simulink model "mech_motorcycle_stability"  (Simulink 7.1)
settings: Solver=ode45  StartTime=0.0  StopTime=3  RelTol=1e-3  AbsTol=1e-6
PreLoadFcn:
  | vu=53;mech_motorcycle_data
values from neighbouring files (symbols this model uses):
  Cf1 = -13.25+1.302*Zf-(1.39e-4)*Zf^2    [mech_motorcycle_data.m]
  Cf2 = 2.788+0.0165*Zf+(3.9e-6)*Zf^2    [mech_motorcycle_data.m]
  Cf3 = -0.06*Zf    [mech_motorcycle_data.m]
  Cfvf = -300+28.577*Zf-0.0143*Zf^2+(1.431e-6)*Zf^3+(3.347e-10)*Zf^4    [mech_motorcycle_data.m]
  Cfvr = -92.9+23.129*Zr-(4.663/1000)*Zr^2-(6.457e-7)*Zr^3+(1.887e-10)*Zr^4    [mech_motorcycle_data.m]
  Cmvf = -0.281+0.2442*Zf+(8.575e-5)*Zf^2    [mech_motorcycle_data.m]
  Cmvr = 9+0.3573*Zr + (3.378e-5)*Zr^2    [mech_motorcycle_data.m]
  Cr1 = 27.38+0.9727*Zr-(4e-6)*Zr^2    [mech_motorcycle_data.m]
  Cr2 = 2.056+0.01282*Zr+(4.928e-6)*Zr^2    [mech_motorcycle_data.m]
  Cr3 = -0.07*Zr    [mech_motorcycle_data.m]
  D = inv(D)    [mech_stewart_MV_controller.m]    (also in mech_stewart_control_Hinf.mat = [-0.999999999853 7.5115525316e-12 1.21216792902e-05 1.919374)
  epsilon = 0.47    [mech_motorcycle_data.m]    (also in mech_motorcycle_data_nonlinear.m = 0.52)
  epsilon1 = 1.435    [mech_motorcycle_data.m]
  G = 9.81    [mech_motorcycle_data.m]    (also in mech_sceng_init.m = 1.4)
  Mfw = 0    [mech_motorcycle_data.m]    (also in mech_motorcycle_data_nonlinear.m = 25.6)
  Mrw = 0    [mech_motorcycle_data.m]    (also in mech_motorcycle_data_nonlinear.m = 25.6)
  Rf = 0.336    [mech_motorcycle_data.m]
  Rr = 0.321    [mech_motorcycle_data.m]
  sigmaf = 0.1012+(1.297e-4)*Zf-(3.267e-8)*Zf^2    [mech_motorcycle_data.m]
  sigmar = 0.03594+(1.941e-4)*Zr-(5.667e-8)*Zr^2+(5.728e-12)*Zr^3    [mech_motorcycle_data.m]
  Zf = ((Mf.value*(bb+kk)+Mr.value*bb+Mb.value*(bb-bb_b)+Mp.value*(bb-bb_p))*G-(vu^2)*(Dc.value*hh_cp+Lc.value*whl_bs/2))/whl_bs    [mech_motorcycle_data.m]
  Zr = (Mf.value+Mr.value+Mp.value+Mb.value)*G-Lc.value*vu^2-Zf    [mech_motorcycle_data.m]
undefined symbols (not defined in the file or in its folder): Crr1, Crr2, D_gamma, D_lamda, D_steer, D_v, D_zita, Dc, ifwy, Ifx, Ifxz, Ifz, Ipx, Ipxz, Ipz, irwx, irwy, Irx, Irxz, iry, Irz, k_gamma, k_lamda, k_steer, k_v, k_zita, Lc, m, Mb, Mf, Mp, Mr, rad, s
libraries: mblibv1 x43
(part 2 of 2)

== system mech_motorcycle_stability/Twist spring-damper ==
  note: Twist spring damper model
  note: Press any key to continue
  Damping : Gain  Gain=-D_lamda.value  ParameterDataType=sfix(16)  ParameterScaling=2^0  OutDataType=sfix(16)  OutScaling=2^0  SaturateOnIntegerOverflow=on  OutDataTypeStr=Inherit: Same as input  ParamDataTypeStr=Inherit: Same as input
  Demux : Demux  Outputs=2
  Initial Force : Constant  Value=0  OutDataType=sfix(16)  OutScaling=2^0
  Joint Actuator : mblibv1/Sensors &  Actuators/Joint Actuator  DialogController=MECH.DynMechDlgSource  SystemSampleTime=-1  PhysicalDomain=Mechanical  PortType=blob  ActuationStyle=Force  AngleUnits=rad  ArcVelocityUnits=rad/s  ArcAccelerationUnits=rad/s^2  CoordPositionUnits=m  VelocityUnits=m/s  AccelerationUnits=m/s^2  ForceUnits=N  TorqueUnits=N-m  ActiveIO=on  Width=1  DialogClass=MechanicalActuatorBlock  Primitive=R1  ReferenceFrame=Absolute (INERTIAL)
  Joint Sensor : mblibv1/Sensors &  Actuators/Joint Sensor  DialogController=MECH.DynMechDlgSource  SystemSampleTime=-1  PhysicalDomain=Mechanical  PortType=blob  Muxed=on  Pose=off  Angle=on  AngleUnits=rad  ArcVelocity=on  ArcVelocityUnits=rad/s  ArcAcceleration=off  ArcAccelerationUnits=deg/s^2  CoordPosition=on  CoordPositionUnits=m  Velocity=on  VelocityUnits=m/s  Acceleration=off  AccelerationUnits=m/s^2  Quaternion=on  QuaternionDT=off  QuaternionDDT=off  QuaternionUnits=off  OutputVector=[ 1 1 ]  ActiveIO=on  Width=2  DialogClass=MechanicalSensorBlock  Primitive=R1  Force=off  ForceUnits=N  Torque=off  TorqueUnits=N-m  ReferenceFrame=Absolute (INERTIAL)  ReactionSensedSide=Base  ReactionReferenceFrame=Absolute (World)  ReactionForce=off  ReactionForceUnits=N  ReactionMoment=off  ReactionMomentUnits=N-m
  Stiffness : Gain  Gain=-k_lamda.value  ParameterDataType=sfix(16)  ParameterScaling=2^0  OutDataType=sfix(16)  OutScaling=2^0  SaturateOnIntegerOverflow=on  OutDataTypeStr=Inherit: Same as input  ParamDataTypeStr=Inherit: Same as input
  Sum : Sum  Inputs=+++  OutDataType=sfix(16)  OutScaling=2^0  SaturateOnIntegerOverflow=on  InputSameDT=on  OutDataTypeStr=Inherit: Same as first input
  S : PMIOPort  Port=1  Side=Left
  A : PMIOPort  Orientation=left  Port=2  Side=Right
  wires:
  Sum/1 -> Joint Actuator/1  "Torque (Nm)"
  Joint Sensor/1 -> Demux/1
  Demux/1 -> Stiffness/1  "Angle (rad)"
  Demux/2 -> Damping/1  "Angular velocity (rad/s)"
  Damping/1 -> Sum/2
  Stiffness/1 -> Sum/1
  Initial Force/1 -> Sum/3
  connections:
  S/RConn1 -- Joint Sensor/LConn1
  Joint Actuator/RConn1 -- A/RConn1

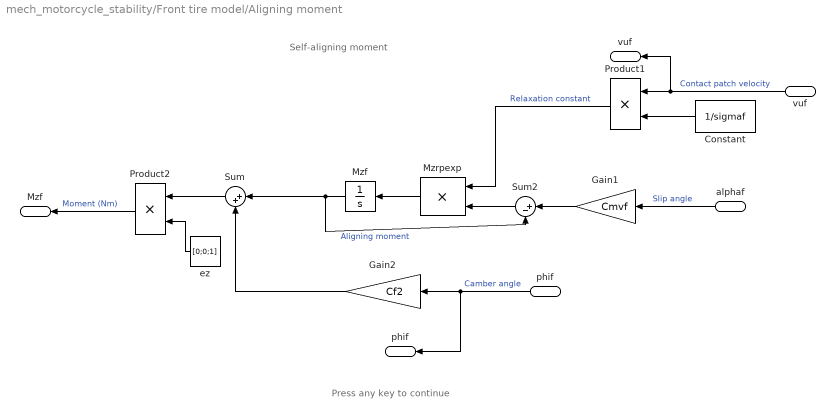
== system mech_motorcycle_stability/Front tire model/Aligning moment ==
  note: Self-aligning moment
  note: Press any key to continue
  vuf : Inport  Orientation=left  OutDataType=sfix(16)  OutScaling=2^0
  phif : Inport  Orientation=left  Port=2  OutDataType=sfix(16)  OutScaling=2^0
  alphaf : Inport  Orientation=left  Port=3  OutDataType=sfix(16)  OutScaling=2^0
  Constant : Constant  Orientation=left  Value=1/sigmaf  OutDataType=sfix(16)  OutScaling=2^0
  Gain1 : Gain  Orientation=left  Gain=Cmvf  ParameterDataType=sfix(16)  ParameterScaling=2^0  OutDataType=sfix(16)  OutScaling=2^0  SaturateOnIntegerOverflow=on  OutDataTypeStr=Inherit: Same as input  ParamDataTypeStr=Inherit: Same as input
  Gain2 : Gain  Orientation=left  Gain=Cf2  ParameterDataType=sfix(16)  ParameterScaling=2^0  OutDataType=sfix(16)  OutScaling=2^0  SaturateOnIntegerOverflow=on  OutDataTypeStr=Inherit: Same as input  ParamDataTypeStr=Inherit: Same as input
  "Mzf  " : Integrator  Orientation=left  ZeroCross=off
  Mzrpexp : Product  Orientation=left  OutDataType=sfix(16)  OutScaling=2^0  SaturateOnIntegerOverflow=on  InputSameDT=on  OutDataTypeStr=Inherit: Same as first input
  Product1 : Product  Orientation=left  OutDataType=sfix(16)  OutScaling=2^0  SaturateOnIntegerOverflow=on  InputSameDT=on  OutDataTypeStr=Inherit: Same as first input
  Product2 : Product  Orientation=left  OutDataType=sfix(16)  OutScaling=2^0  SaturateOnIntegerOverflow=on  InputSameDT=on  OutDataTypeStr=Inherit: Same as first input
  Sum : Sum  Orientation=left  Inputs=|++  OutDataType=sfix(16)  OutScaling=2^0  SaturateOnIntegerOverflow=on  InputSameDT=on  OutDataTypeStr=Inherit: Same as first input
  Sum2 : Sum  Orientation=left  Inputs=|+-  OutDataType=sfix(16)  OutScaling=2^0  SaturateOnIntegerOverflow=on  InputSameDT=on  OutDataTypeStr=Inherit: Same as first input
  ez : Constant  Orientation=left  Value=[0;0;1]  OutDataType=sfix(16)  OutScaling=2^0
  Mzf : Outport  Orientation=left  OutDataType=sfix(16)  OutScaling=2^0
  "phif " : Outport  Orientation=left  Port=2  OutDataType=sfix(16)  OutScaling=2^0
  "vuf " : Outport  Orientation=left  Port=3  OutDataType=sfix(16)  OutScaling=2^0
  wires:
  Product2/1 -> Mzf/1  "Moment (Nm)"
  ez/1 -> Product2/2
  Sum/1 -> Product2/1
  Gain2/1 -> Sum/2
  phif/1 -> "phif "/1, Gain2/1  "Camber angle"
  alphaf/1 -> Gain1/1  "Slip angle"
  "Mzf  "/1 -> Sum2/2, Sum/1  "Aligning moment"
  Gain1/1 -> Sum2/1
  Sum2/1 -> Mzrpexp/2
  Product1/1 -> Mzrpexp/1  "Relaxation constant"
  Mzrpexp/1 -> "Mzf  "/1
  Constant/1 -> Product1/2
  vuf/1 -> Product1/1, "vuf "/1  "Contact patch velocity"

== system mech_motorcycle_stability/Front tire model/Contact ==
  note: Contact
  note: Press any key to continue
  Body Sensor : mblibv1/Sensors &  Actuators/Body Sensor  Orientation=left  DialogController=MECH.DynMechDlgSource  SystemSampleTime=-1  PhysicalDomain=Mechanical  PortType=blob  Muxed=off  Pose=on  Angle=on  AngleUnits=deg  ArcVelocity=off  ArcVelocityUnits=rad/s  ArcAcceleration=off  ArcAccelerationUnits=rad/s^2  CoordPosition=off  CoordPositionUnits=m  Velocity=on  VelocityUnits=m/s  Acceleration=off  AccelerationUnits=m/s^2  Quaternion=on  QuaternionDT=off  QuaternionDDT=off  QuaternionUnits=off  OutputVector=[ 3 9 ]  ActiveIO=on  Width=12  DialogClass=MechanicalSensorBlock  ReferenceFrame=Absolute (World)
  Contact geometry : Subsystem  Orientation=left
  Product1 : Product  Orientation=left  Multiplication=Matrix(*)  OutDataType=sfix(16)  OutScaling=2^0  SaturateOnIntegerOverflow=on  InputSameDT=on  OutDataTypeStr=Inherit: Same as first input
  Reshape : Reshape  Orientation=left  OutputDimensionality=Row vector (2-D)
  Reshape1 : Reshape  Orientation=left  OutputDimensionality=Column vector (2-D)
  Rear Wheel : PMIOPort  Orientation=left  Port=1  Side=Left
  fw_long : Outport  Orientation=left  OutDataType=sfix(16)  OutScaling=2^0
  vuf : Outport  Orientation=left  Port=2  OutDataType=sfix(16)  OutScaling=2^0
  phif : Outport  Orientation=left  Port=3  OutDataType=sfix(16)  OutScaling=2^0
  dfwcp_dt : Outport  Orientation=left  Port=4  OutDataType=sfix(16)  OutScaling=2^0
  fw_lat : Outport  Orientation=left  Port=5  OutDataType=sfix(16)  OutScaling=2^0
  wires:
  Contact geometry/3(phif) -> phif/1  "Camber angle (rad)"
  Contact geometry/1(fw_lat) -> fw_lat/1  "Lateral direction"
  Body Sensor/2 -> Contact geometry/1(T)  "Body orientation"
  Reshape1/1 -> Product1/2
  Reshape/1 -> Product1/1
  Product1/1 -> vuf/1  "Longitudinal component (m/s)"
  Body Sensor/1 -> Reshape/1, dfwcp_dt/1  "Contact patch velocity (m/s)"
  Contact geometry/2(fw_long) -> fw_long/1, Reshape1/1  "Longitudinal direction"
  connections:
  Rear Wheel/RConn1 -- Body Sensor/LConn1

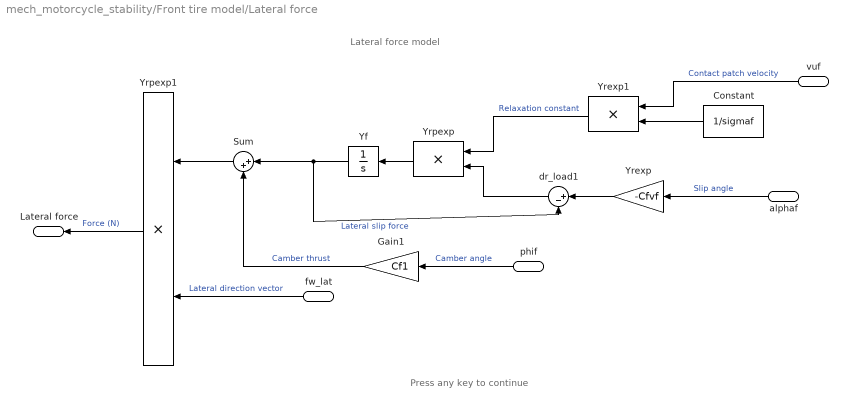
== system mech_motorcycle_stability/Front tire model/Lateral force ==
  note: Lateral force model
  note: Press any key to continue
  phif : Inport  Orientation=left  OutDataType=sfix(16)  OutScaling=2^0
  vuf : Inport  Orientation=left  Port=2  OutDataType=sfix(16)  OutScaling=2^0
  alphaf : Inport  Orientation=left  Port=3  OutDataType=sfix(16)  OutScaling=2^0
  fw_lat : Inport  Orientation=left  Port=4  OutDataType=sfix(16)  OutScaling=2^0
  Constant : Constant  Orientation=left  Value=1/sigmaf  OutDataType=sfix(16)  OutScaling=2^0
  Gain1 : Gain  Orientation=left  Gain=Cf1  ParameterDataType=sfix(16)  ParameterScaling=2^0  OutDataType=sfix(16)  OutScaling=2^0  SaturateOnIntegerOverflow=on  OutDataTypeStr=Inherit: Same as input  ParamDataTypeStr=Inherit: Same as input
  Sum : Sum  Orientation=left  Inputs=|++  OutDataType=sfix(16)  OutScaling=2^0  SaturateOnIntegerOverflow=on  InputSameDT=on  OutDataTypeStr=Inherit: Same as first input
  Yf : Integrator  Orientation=left  ZeroCross=off
  Yrexp : Gain  Orientation=left  Gain=-Cfvf  ParameterDataType=sfix(16)  ParameterScaling=2^0  OutDataType=sfix(16)  OutScaling=2^0  SaturateOnIntegerOverflow=on  OutDataTypeStr=Inherit: Same as input  ParamDataTypeStr=Inherit: Same as input
  Yrexp1 : Product  Orientation=left  OutDataType=sfix(16)  OutScaling=2^0  SaturateOnIntegerOverflow=on  InputSameDT=on  OutDataTypeStr=Inherit: Same as first input
  Yrpexp : Product  Orientation=left  OutDataType=sfix(16)  OutScaling=2^0  SaturateOnIntegerOverflow=on  InputSameDT=on  OutDataTypeStr=Inherit: Same as first input
  Yrpexp1 : Product  Orientation=left  OutDataType=sfix(16)  OutScaling=2^0  SaturateOnIntegerOverflow=on  InputSameDT=on  OutDataTypeStr=Inherit: Same as first input
  dr_load1 : Sum  Orientation=left  Inputs=|+-  OutDataType=sfix(16)  OutScaling=2^0  SaturateOnIntegerOverflow=on  InputSameDT=on  OutDataTypeStr=Inherit: Same as first input
  Lateral force : Outport  Orientation=left  OutDataType=sfix(16)  OutScaling=2^0
  wires:
  Yrpexp1/1 -> Lateral force/1  "Force (N)"
  fw_lat/1 -> Yrpexp1/2  "Lateral direction vector"
  Sum/1 -> Yrpexp1/1
  Gain1/1 -> Sum/2  "Camber thrust"
  phif/1 -> Gain1/1  "Camber angle"
  alphaf/1 -> Yrexp/1  "Slip angle"
  Yrexp/1 -> dr_load1/1
  Yf/1 -> Sum/1, dr_load1/2  "Lateral slip force"
  Yrpexp/1 -> Yf/1
  dr_load1/1 -> Yrpexp/2
  Yrexp1/1 -> Yrpexp/1  "Relaxation constant"
  Constant/1 -> Yrexp1/2
  vuf/1 -> Yrexp1/1  "Contact patch velocity"

== system mech_motorcycle_stability/Front tire model/Lateral slip computation ==
  note: Lateral slip computation
  note: Press any key to continue
  dfwcp_dt : Inport  Orientation=left  OutDataType=sfix(16)  OutScaling=2^0
  fw_lat : Inport  Orientation=left  Port=2  OutDataType=sfix(16)  OutScaling=2^0
  Fcn : Fcn  Orientation=left  Expr=1.0/sqrt(u[1]*u[1] + u[2]*u[2] + u[3]*u[3])
  Product : Product  Orientation=left  OutDataType=sfix(16)  OutScaling=2^0  SaturateOnIntegerOverflow=on  InputSameDT=on  OutDataTypeStr=Inherit: Same as first input
  Product1 : Product  Orientation=left  Multiplication=Matrix(*)  OutDataType=sfix(16)  OutScaling=2^0  SaturateOnIntegerOverflow=on  InputSameDT=on  OutDataTypeStr=Inherit: Same as first input
  Reshape : Reshape  Orientation=left  OutputDimensionality=Row vector (2-D)
  Reshape1 : Reshape  Orientation=left  OutputDimensionality=Column vector (2-D)
  Trigonometric Function : Trigonometry  Orientation=left  Operator=asin
  alphaf : Outport  Orientation=left  OutDataType=sfix(16)  OutScaling=2^0
  wires:
  Product/1 -> Reshape/1  "Unit vector"
  Fcn/1 -> Product/1
  dfwcp_dt/1 -> Fcn/1, Product/2  "Velocity (m/s)"
  fw_lat/1 -> Reshape1/1  "Lateral direction"
  Reshape1/1 -> Product1/2
  Trigonometric Function/1 -> alphaf/1  "Slip angle (rad)"
  Product1/1 -> Trigonometric Function/1
  Reshape/1 -> Product1/1

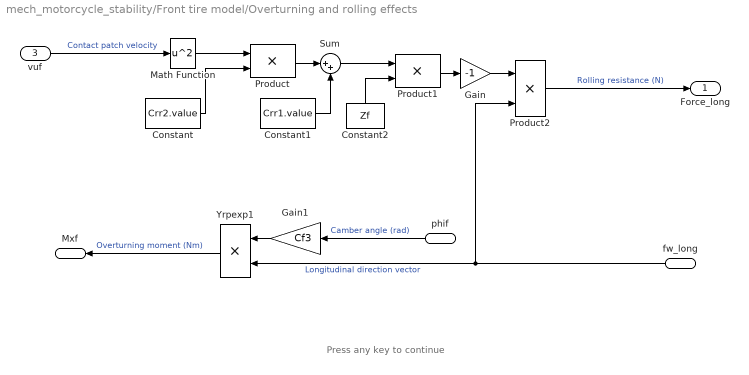
== system mech_motorcycle_stability/Front tire model/Overturning and rolling effects ==
  note: Press any key to continue
  fw_long : Inport  Orientation=left  OutDataType=sfix(16)  OutScaling=2^0
  phif : Inport  Orientation=left  Port=2  OutDataType=sfix(16)  OutScaling=2^0
  vuf : Inport  Port=3  OutDataType=sfix(16)  OutScaling=2^0
  Constant : Constant  Value=Crr2.value  OutDataType=sfix(16)  OutScaling=2^0
  Constant1 : Constant  Value=Crr1.value  OutDataType=sfix(16)  OutScaling=2^0
  Constant2 : Constant  Orientation=up  Value=Zf  OutDataType=sfix(16)  OutScaling=2^0
  Gain : Gain  Gain=-1  ParameterDataType=sfix(16)  ParameterScaling=2^0  OutDataType=sfix(16)  OutScaling=2^0  SaturateOnIntegerOverflow=on  OutDataTypeStr=Inherit: Same as input  ParamDataTypeStr=Inherit: Same as input
  Gain1 : Gain  Orientation=left  Gain=Cf3  ParameterDataType=sfix(16)  ParameterScaling=2^0  OutDataType=sfix(16)  OutScaling=2^0  SaturateOnIntegerOverflow=on  OutDataTypeStr=Inherit: Same as input  ParamDataTypeStr=Inherit: Same as input
  Math Function : Math  Operator=square  OutDataType=sfix(16)  OutScaling=2^0  SaturateOnIntegerOverflow=on
  Product : Product  OutDataType=sfix(16)  OutScaling=2^0  SaturateOnIntegerOverflow=on  InputSameDT=on  OutDataTypeStr=Inherit: Same as first input
  Product1 : Product  OutDataType=sfix(16)  OutScaling=2^0  SaturateOnIntegerOverflow=on  InputSameDT=on  OutDataTypeStr=Inherit: Same as first input
  Product2 : Product  OutDataType=sfix(16)  OutScaling=2^0  SaturateOnIntegerOverflow=on  InputSameDT=on  OutDataTypeStr=Inherit: Same as first input
  Sum : Sum  Inputs=|++  OutDataType=sfix(16)  OutScaling=2^0  SaturateOnIntegerOverflow=on  InputSameDT=on  OutDataTypeStr=Inherit: Same as first input
  Yrpexp1 : Product  Orientation=left  OutDataType=sfix(16)  OutScaling=2^0  SaturateOnIntegerOverflow=on  InputSameDT=on  OutDataTypeStr=Inherit: Same as first input
  Force_long : Outport  OutDataType=sfix(16)  OutScaling=2^0
  Mxf : Outport  Orientation=left  Port=2  OutDataType=sfix(16)  OutScaling=2^0
  wires:
  Yrpexp1/1 -> Mxf/1  "Overturning moment (Nm)"
  Gain1/1 -> Yrpexp1/1
  phif/1 -> Gain1/1  "Camber angle (rad)"
  Product2/1 -> Force_long/1  "Rolling resistance (N)"
  Gain/1 -> Product2/1
  Product1/1 -> Gain/1
  Constant2/1 -> Product1/2
  Sum/1 -> Product1/1
  Constant1/1 -> Sum/2
  Constant/1 -> Product/2
  Math Function/1 -> Product/1
  Product/1 -> Sum/1
  vuf/1 -> Math Function/1  "Contact patch velocity"
  fw_long/1 -> Yrpexp1/2, Product2/2  "Longitudinal direction vector"

== system mech_motorcycle_stability/Front tire model/Vertical force ==
  note: Press any key to continue
  Constant : Constant  Orientation=left  Value=-Zf  OutDataType=sfix(16)  OutScaling=2^0
  Product2 : Product  Orientation=left  OutDataType=sfix(16)  OutScaling=2^0  SaturateOnIntegerOverflow=on  InputSameDT=on  OutDataTypeStr=Inherit: Same as first input
  ez : Constant  Orientation=left  Value=[0;0;1]  OutDataType=sfix(16)  OutScaling=2^0
  Force_vert : Outport  Orientation=left  OutDataType=sfix(16)  OutScaling=2^0
  wires:
  ez/1 -> Product2/2
  Constant/1 -> Product2/1
  Product2/1 -> Force_vert/1  "Vertical force (N)"

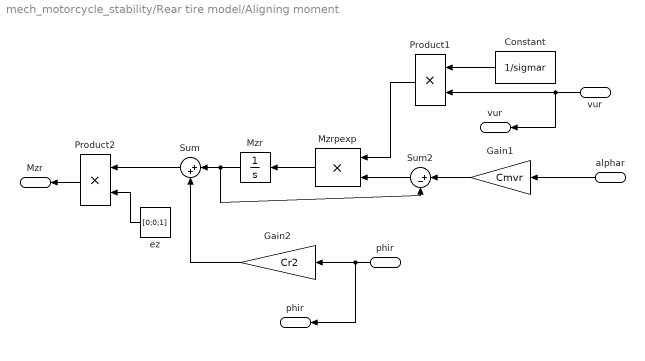
== system mech_motorcycle_stability/Rear tire model/Aligning moment ==
  vur : Inport  Orientation=left  OutDataType=sfix(16)  OutScaling=2^0
  phir : Inport  Orientation=left  Port=2  OutDataType=sfix(16)  OutScaling=2^0
  alphar : Inport  Orientation=left  Port=3  OutDataType=sfix(16)  OutScaling=2^0
  Constant : Constant  Orientation=left  Value=1/sigmar  OutDataType=sfix(16)  OutScaling=2^0
  Gain1 : Gain  Orientation=left  Gain=Cmvr  ParameterDataType=sfix(16)  ParameterScaling=2^0  OutDataType=sfix(16)  OutScaling=2^0  SaturateOnIntegerOverflow=on  OutDataTypeStr=Inherit: Same as input  ParamDataTypeStr=Inherit: Same as input
  Gain2 : Gain  Orientation=left  Gain=Cr2  ParameterDataType=sfix(16)  ParameterScaling=2^0  OutDataType=sfix(16)  OutScaling=2^0  SaturateOnIntegerOverflow=on  OutDataTypeStr=Inherit: Same as input  ParamDataTypeStr=Inherit: Same as input
  "Mzr  " : Integrator  Orientation=left  ZeroCross=off
  Mzrpexp : Product  Orientation=left  OutDataType=sfix(16)  OutScaling=2^0  SaturateOnIntegerOverflow=on  InputSameDT=on  OutDataTypeStr=Inherit: Same as first input
  Product1 : Product  Orientation=left  OutDataType=sfix(16)  OutScaling=2^0  SaturateOnIntegerOverflow=on  InputSameDT=on  OutDataTypeStr=Inherit: Same as first input
  Product2 : Product  Orientation=left  OutDataType=sfix(16)  OutScaling=2^0  SaturateOnIntegerOverflow=on  InputSameDT=on  OutDataTypeStr=Inherit: Same as first input
  Sum : Sum  Orientation=left  Inputs=|++  OutDataType=sfix(16)  OutScaling=2^0  SaturateOnIntegerOverflow=on  InputSameDT=on  OutDataTypeStr=Inherit: Same as first input
  Sum2 : Sum  Orientation=left  Inputs=|+-  OutDataType=sfix(16)  OutScaling=2^0  SaturateOnIntegerOverflow=on  InputSameDT=on  OutDataTypeStr=Inherit: Same as first input
  ez : Constant  Orientation=left  Value=[0;0;1]  OutDataType=sfix(16)  OutScaling=2^0
  Mzr : Outport  Orientation=left  OutDataType=sfix(16)  OutScaling=2^0
  "phir " : Outport  Orientation=left  Port=2  OutDataType=sfix(16)  OutScaling=2^0
  "vur " : Outport  Orientation=left  Port=3  OutDataType=sfix(16)  OutScaling=2^0
  wires:
  Mzrpexp/1 -> "Mzr  "/1
  Product1/1 -> Mzrpexp/1
  Sum2/1 -> Mzrpexp/2
  vur/1 -> Product1/2, "vur "/1
  Gain1/1 -> Sum2/1
  "Mzr  "/1 -> Sum2/2, Sum/1
  alphar/1 -> Gain1/1
  Constant/1 -> Product1/1
  phir/1 -> Gain2/1, "phir "/1
  Gain2/1 -> Sum/2
  Sum/1 -> Product2/1
  ez/1 -> Product2/2
  Product2/1 -> Mzr/1

== system mech_motorcycle_stability/Rear tire model/Contact ==
  Body Sensor : mblibv1/Sensors &  Actuators/Body Sensor  Orientation=left  DialogController=MECH.DynMechDlgSource  SystemSampleTime=-1  PhysicalDomain=Mechanical  PortType=blob  Muxed=off  Pose=on  Angle=on  AngleUnits=deg  ArcVelocity=off  ArcVelocityUnits=rad/s  ArcAcceleration=off  ArcAccelerationUnits=rad/s^2  CoordPosition=off  CoordPositionUnits=m  Velocity=on  VelocityUnits=m/s  Acceleration=off  AccelerationUnits=m/s^2  Quaternion=on  QuaternionDT=off  QuaternionDDT=off  QuaternionUnits=off  OutputVector=[ 3 9 ]  ActiveIO=on  Width=12  DialogClass=MechanicalSensorBlock  ReferenceFrame=Absolute (World)
  Contact geometry : Subsystem  Orientation=left
  Product1 : Product  Orientation=left  Multiplication=Matrix(*)  OutDataType=sfix(16)  OutScaling=2^0  SaturateOnIntegerOverflow=on  InputSameDT=on  OutDataTypeStr=Inherit: Same as first input
  Reshape : Reshape  Orientation=left  OutputDimensionality=Row vector (2-D)
  Reshape1 : Reshape  Orientation=left  OutputDimensionality=Column vector (2-D)
  Rear Wheel : PMIOPort  Orientation=left  Port=1  Side=Left
  rw_long : Outport  Orientation=left  OutDataType=sfix(16)  OutScaling=2^0
  vur : Outport  Orientation=left  Port=2  OutDataType=sfix(16)  OutScaling=2^0
  phir : Outport  Orientation=left  Port=3  OutDataType=sfix(16)  OutScaling=2^0
  drwcp_dt : Outport  Orientation=left  Port=4  OutDataType=sfix(16)  OutScaling=2^0
  rw_lat : Outport  Orientation=left  Port=5  OutDataType=sfix(16)  OutScaling=2^0
  wires:
  Body Sensor/2 -> Contact geometry/1(T)
  Contact geometry/1(rw_lat) -> rw_lat/1
  Contact geometry/3(phir) -> phir/1
  Reshape1/1 -> Product1/2
  Reshape/1 -> Product1/1
  Product1/1 -> vur/1
  Body Sensor/1 -> Reshape/1, drwcp_dt/1
  Contact geometry/2(rw_long) -> rw_long/1, Reshape1/1
  connections:
  Rear Wheel/RConn1 -- Body Sensor/LConn1

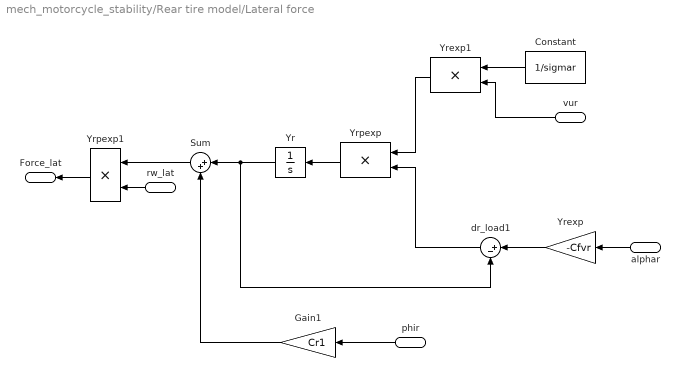
== system mech_motorcycle_stability/Rear tire model/Lateral force ==
  phir : Inport  Orientation=left  OutDataType=sfix(16)  OutScaling=2^0
  vur : Inport  Orientation=left  Port=2  OutDataType=sfix(16)  OutScaling=2^0
  alphar : Inport  Orientation=left  Port=3  OutDataType=sfix(16)  OutScaling=2^0
  rw_lat : Inport  Orientation=left  Port=4  OutDataType=sfix(16)  OutScaling=2^0
  Constant : Constant  Orientation=left  Value=1/sigmar  OutDataType=sfix(16)  OutScaling=2^0
  Gain1 : Gain  Orientation=left  Gain=Cr1  ParameterDataType=sfix(16)  ParameterScaling=2^0  OutDataType=sfix(16)  OutScaling=2^0  SaturateOnIntegerOverflow=on  OutDataTypeStr=Inherit: Same as input  ParamDataTypeStr=Inherit: Same as input
  Sum : Sum  Orientation=left  Inputs=|++  OutDataType=sfix(16)  OutScaling=2^0  SaturateOnIntegerOverflow=on  InputSameDT=on  OutDataTypeStr=Inherit: Same as first input
  Yr : Integrator  Orientation=left  ZeroCross=off
  Yrexp : Gain  Orientation=left  Gain=-Cfvr  ParameterDataType=sfix(16)  ParameterScaling=2^0  OutDataType=sfix(16)  OutScaling=2^0  SaturateOnIntegerOverflow=on  OutDataTypeStr=Inherit: Same as input  ParamDataTypeStr=Inherit: Same as input
  Yrexp1 : Product  Orientation=left  OutDataType=sfix(16)  OutScaling=2^0  SaturateOnIntegerOverflow=on  InputSameDT=on  OutDataTypeStr=Inherit: Same as first input
  Yrpexp : Product  Orientation=left  OutDataType=sfix(16)  OutScaling=2^0  SaturateOnIntegerOverflow=on  InputSameDT=on  OutDataTypeStr=Inherit: Same as first input
  Yrpexp1 : Product  Orientation=left  OutDataType=sfix(16)  OutScaling=2^0  SaturateOnIntegerOverflow=on  InputSameDT=on  OutDataTypeStr=Inherit: Same as first input
  dr_load1 : Sum  Orientation=left  Inputs=|+-  OutDataType=sfix(16)  OutScaling=2^0  SaturateOnIntegerOverflow=on  InputSameDT=on  OutDataTypeStr=Inherit: Same as first input
  Force_lat : Outport  Orientation=left  OutDataType=sfix(16)  OutScaling=2^0
  wires:
  Yrexp1/1 -> Yrpexp/1
  dr_load1/1 -> Yrpexp/2
  Yrpexp/1 -> Yr/1
  Yr/1 -> dr_load1/2, Sum/1
  vur/1 -> Yrexp1/2
  Yrexp/1 -> dr_load1/1
  alphar/1 -> Yrexp/1
  Constant/1 -> Yrexp1/1
  phir/1 -> Gain1/1
  Gain1/1 -> Sum/2
  Sum/1 -> Yrpexp1/1
  rw_lat/1 -> Yrpexp1/2
  Yrpexp1/1 -> Force_lat/1

== system mech_motorcycle_stability/Rear tire model/Lateral slip computation ==
  drwcp_dt : Inport  Orientation=left  OutDataType=sfix(16)  OutScaling=2^0
  rw_lat : Inport  Orientation=left  Port=2  OutDataType=sfix(16)  OutScaling=2^0
  Fcn : Fcn  Orientation=left  Expr=1.0/sqrt(u[1]*u[1] + u[2]*u[2] + u[3]*u[3])
  Product : Product  Orientation=left  OutDataType=sfix(16)  OutScaling=2^0  SaturateOnIntegerOverflow=on  InputSameDT=on  OutDataTypeStr=Inherit: Same as first input
  Product1 : Product  Orientation=left  Multiplication=Matrix(*)  OutDataType=sfix(16)  OutScaling=2^0  SaturateOnIntegerOverflow=on  InputSameDT=on  OutDataTypeStr=Inherit: Same as first input
  Reshape : Reshape  Orientation=left  OutputDimensionality=Row vector (2-D)
  Reshape1 : Reshape  Orientation=left  OutputDimensionality=Column vector (2-D)
  Trigonometric Function : Trigonometry  Orientation=left  Operator=asin
  alphar : Outport  Orientation=left  OutDataType=sfix(16)  OutScaling=2^0
  wires:
  Reshape/1 -> Product1/1
  Product1/1 -> Trigonometric Function/1
  Trigonometric Function/1 -> alphar/1
  Reshape1/1 -> Product1/2
  rw_lat/1 -> Reshape1/1
  drwcp_dt/1 -> Product/2, Fcn/1
  Fcn/1 -> Product/1
  Product/1 -> Reshape/1

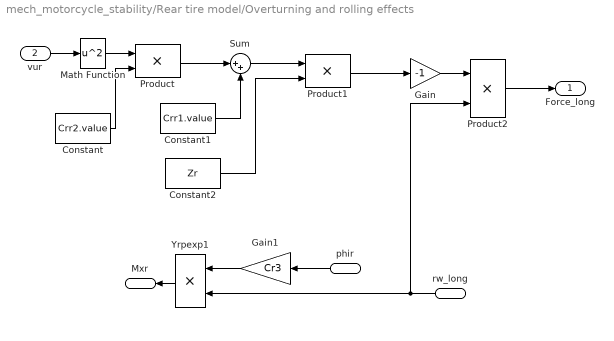
== system mech_motorcycle_stability/Rear tire model/Overturning and rolling effects ==
  rw_long : Inport  Orientation=left  OutDataType=sfix(16)  OutScaling=2^0
  vur : Inport  Port=2  OutDataType=sfix(16)  OutScaling=2^0
  phir : Inport  Orientation=left  Port=3  OutDataType=sfix(16)  OutScaling=2^0
  Constant : Constant  Value=Crr2.value  OutDataType=sfix(16)  OutScaling=2^0
  Constant1 : Constant  Value=Crr1.value  OutDataType=sfix(16)  OutScaling=2^0
  Constant2 : Constant  Value=Zr  OutDataType=sfix(16)  OutScaling=2^0
  Gain : Gain  Gain=-1  ParameterDataType=sfix(16)  ParameterScaling=2^0  OutDataType=sfix(16)  OutScaling=2^0  SaturateOnIntegerOverflow=on  OutDataTypeStr=Inherit: Same as input  ParamDataTypeStr=Inherit: Same as input
  Gain1 : Gain  Orientation=left  Gain=Cr3  ParameterDataType=sfix(16)  ParameterScaling=2^0  OutDataType=sfix(16)  OutScaling=2^0  SaturateOnIntegerOverflow=on  OutDataTypeStr=Inherit: Same as input  ParamDataTypeStr=Inherit: Same as input
  Math Function : Math  Operator=square  OutDataType=sfix(16)  OutScaling=2^0  SaturateOnIntegerOverflow=on
  Product : Product  OutDataType=sfix(16)  OutScaling=2^0  SaturateOnIntegerOverflow=on  InputSameDT=on  OutDataTypeStr=Inherit: Same as first input
  Product1 : Product  OutDataType=sfix(16)  OutScaling=2^0  SaturateOnIntegerOverflow=on  InputSameDT=on  OutDataTypeStr=Inherit: Same as first input
  Product2 : Product  OutDataType=sfix(16)  OutScaling=2^0  SaturateOnIntegerOverflow=on  InputSameDT=on  OutDataTypeStr=Inherit: Same as first input
  Sum : Sum  Inputs=|++  OutDataType=sfix(16)  OutScaling=2^0  SaturateOnIntegerOverflow=on  InputSameDT=on  OutDataTypeStr=Inherit: Same as first input
  Yrpexp1 : Product  Orientation=left  OutDataType=sfix(16)  OutScaling=2^0  SaturateOnIntegerOverflow=on  InputSameDT=on  OutDataTypeStr=Inherit: Same as first input
  Force_long : Outport  OutDataType=sfix(16)  OutScaling=2^0
  Mxr : Outport  Orientation=left  Port=2  OutDataType=sfix(16)  OutScaling=2^0
  wires:
  vur/1 -> Math Function/1
  Product/1 -> Sum/1
  Math Function/1 -> Product/1
  Constant/1 -> Product/2
  Constant1/1 -> Sum/2
  Sum/1 -> Product1/1
  Constant2/1 -> Product1/2
  Product1/1 -> Gain/1
  Gain/1 -> Product2/1
  Product2/1 -> Force_long/1
  phir/1 -> Gain1/1
  Gain1/1 -> Yrpexp1/1
  Yrpexp1/1 -> Mxr/1
  rw_long/1 -> Yrpexp1/2, Product2/2

== system mech_motorcycle_stability/Rear tire model/Vertical force ==
  Constant : Constant  Orientation=left  Value=-Zr  OutDataType=sfix(16)  OutScaling=2^0
  Product2 : Product  Orientation=left  OutDataType=sfix(16)  OutScaling=2^0  SaturateOnIntegerOverflow=on  InputSameDT=on  OutDataTypeStr=Inherit: Same as first input
  ez : Constant  Orientation=left  Value=[0;0;1]  OutDataType=sfix(16)  OutScaling=2^0
  Force_vert : Outport  Orientation=left  OutDataType=sfix(16)  OutScaling=2^0
  wires:
  Product2/1 -> Force_vert/1
  Constant/1 -> Product2/1
  ez/1 -> Product2/2

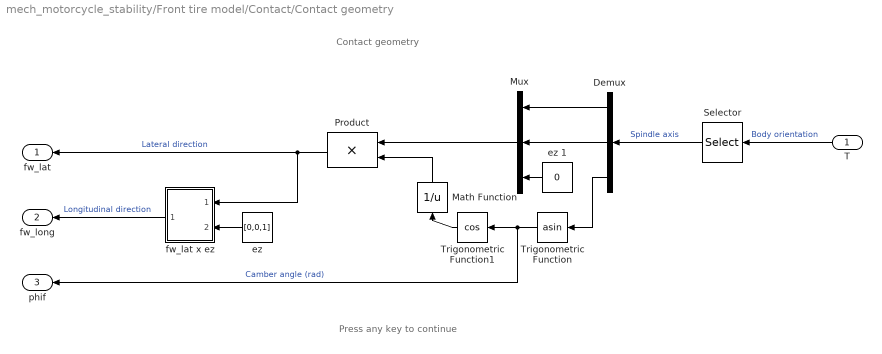
== system mech_motorcycle_stability/Front tire model/Contact/Contact geometry ==
  note: Contact geometry
  note: Press any key to continue
  T : Inport  Orientation=left  OutDataType=sfix(16)  OutScaling=2^0
  Demux : Demux  Orientation=left  Outputs=3
  Math Function : Math  Orientation=up  Operator=reciprocal  OutDataType=sfix(16)  OutScaling=2^0  SaturateOnIntegerOverflow=on
  Mux : Mux  Orientation=left  Inputs=3
  Product : Product  Orientation=left  OutDataType=sfix(16)  OutScaling=2^0  SaturateOnIntegerOverflow=on  InputSameDT=on  OutDataTypeStr=Inherit: Same as first input
  Selector : Selector  Orientation=left  InputPortWidth=9  IndexOptions=Index vector (dialog)  Indices=[4:6]  OutputSizes=1
  Trigonometric Function : Trigonometry  Orientation=left  Operator=asin
  Trigonometric Function1 : Trigonometry  Orientation=left  Operator=cos
  "ez " : Constant  Orientation=left  Value=[0,0,1]  OutDataType=sfix(16)  OutScaling=2^0
  ez 1 : Constant  Orientation=left  Value=0  OutDataType=sfix(16)  OutScaling=2^0
  fw_lat x ez : Subsystem  Orientation=left
      mask Type: Cross Product
      mask Description: Calculates the cross product of two 3x1 vectors.
      mask Help:
      | <p>This block calculates the cross product of two 3x1 vectors, ie.</p>
      | 
      | <ul>C(1) = A(2)*B(3) - A(3)*B(2)</ul>
      | <ul>C(2) = A(3)*B(1) - A(1)*B(3)</ul>
      | <ul>C(3) = A(1)*B(2) - A(2)*B(1)</ul>
      | 
      | <p>The block inputs and output contain more than one signal as described below.</p>
      | 
      | <p><H4>Block Vector Input 1 - A</H4>
      | <ul>
      | <li>A(1)</li>
      | <li>A(2)</li>
      | <li>A(3)</li>
      | </ul>
      | </p>
      | 
      | <p><H4>Block Vector Input 2 - B</H4>
      | <ul>
      | <li>B(1)</li>
      | <li>B(2)</li>
      | <li>B(3)</li>
      | </ul>
      | </p>
      | 
      | <p><H4>Block Vector Output - Cross Product (AxB)</H4>
      | <ul>
      | <li>C(1)</li>
      | <li>C(2)</li>
      | <li>C(3)</li>
      | </ul>
      | </p>
      mask Display: disp('Cross\nProduct')
  fw_lat : Outport  Orientation=left  OutDataType=sfix(16)  OutScaling=2^0
  fw_long : Outport  Orientation=left  Port=2  OutDataType=sfix(16)  OutScaling=2^0
  phif : Outport  Orientation=left  Port=3  OutDataType=sfix(16)  OutScaling=2^0
  wires:
  Selector/1 -> Demux/1  "Spindle axis"
  Product/1 -> fw_lat x ez/1(a(1) a(2) a(3)), fw_lat/1  "Lateral direction"
  Math Function/1 -> Product/2
  Mux/1 -> Product/1
  Demux/3 -> Trigonometric Function/1
  Trigonometric Function1/1 -> Math Function/1
  Trigonometric Function/1 -> Trigonometric Function1/1, phif/1  "Camber angle (rad)"
  T/1 -> Selector/1  "Body orientation"
  ez 1/1 -> Mux/3
  Demux/2 -> Mux/2
  Demux/1 -> Mux/1
  fw_lat x ez/1(c(1) c(2) c(3)) -> fw_long/1  "Longitudinal direction"
  "ez "/1 -> fw_lat x ez/2(b(1) b(2) b(3))

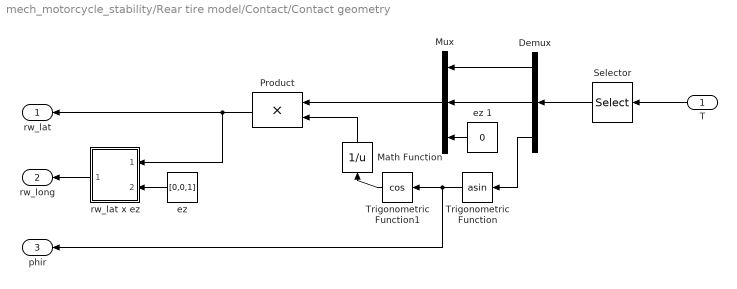
== system mech_motorcycle_stability/Rear tire model/Contact/Contact geometry ==
  T : Inport  Orientation=left  OutDataType=sfix(16)  OutScaling=2^0
  Demux : Demux  Orientation=left  Outputs=3
  Math Function : Math  Orientation=up  Operator=reciprocal  OutDataType=sfix(16)  OutScaling=2^0  SaturateOnIntegerOverflow=on
  Mux : Mux  Orientation=left  Inputs=3
  Product : Product  Orientation=left  OutDataType=sfix(16)  OutScaling=2^0  SaturateOnIntegerOverflow=on  InputSameDT=on  OutDataTypeStr=Inherit: Same as first input
  Selector : Selector  Orientation=left  InputPortWidth=9  IndexOptions=Index vector (dialog)  Indices=[4:6]  OutputSizes=1
  Trigonometric Function : Trigonometry  Orientation=left  Operator=asin
  Trigonometric Function1 : Trigonometry  Orientation=left  Operator=cos
  "ez " : Constant  Orientation=left  Value=[0,0,1]  OutDataType=sfix(16)  OutScaling=2^0
  ez 1 : Constant  Orientation=left  Value=0  OutDataType=sfix(16)  OutScaling=2^0
  rw_lat x ez : Subsystem  Orientation=left
      mask Type: Cross Product
      mask Description: Calculates the cross product of two 3x1 vectors.
      mask Help:
      | <p>This block calculates the cross product of two 3x1 vectors, ie.</p>
      | 
      | <ul>C(1) = A(2)*B(3) - A(3)*B(2)</ul>
      | <ul>C(2) = A(3)*B(1) - A(1)*B(3)</ul>
      | <ul>C(3) = A(1)*B(2) - A(2)*B(1)</ul>
      | 
      | <p>The block inputs and output contain more than one signal as described below.</p>
      | 
      | <p><H4>Block Vector Input 1 - A</H4>
      | <ul>
      | <li>A(1)</li>
      | <li>A(2)</li>
      | <li>A(3)</li>
      | </ul>
      | </p>
      | 
      | <p><H4>Block Vector Input 2 - B</H4>
      | <ul>
      | <li>B(1)</li>
      | <li>B(2)</li>
      | <li>B(3)</li>
      | </ul>
      | </p>
      | 
      | <p><H4>Block Vector Output - Cross Product (AxB)</H4>
      | <ul>
      | <li>C(1)</li>
      | <li>C(2)</li>
      | <li>C(3)</li>
      | </ul>
      | </p>
      mask Display: disp('Cross\nProduct')
  rw_lat : Outport  Orientation=left  OutDataType=sfix(16)  OutScaling=2^0
  rw_long : Outport  Orientation=left  Port=2  OutDataType=sfix(16)  OutScaling=2^0
  phir : Outport  Orientation=left  Port=3  OutDataType=sfix(16)  OutScaling=2^0
  wires:
  "ez "/1 -> rw_lat x ez/2(b(1) b(2) b(3))
  rw_lat x ez/1(c(1) c(2) c(3)) -> rw_long/1
  Demux/1 -> Mux/1
  Demux/2 -> Mux/2
  ez 1/1 -> Mux/3
  T/1 -> Selector/1
  Trigonometric Function/1 -> Trigonometric Function1/1, phir/1
  Trigonometric Function1/1 -> Math Function/1
  Demux/3 -> Trigonometric Function/1
  Mux/1 -> Product/1
  Math Function/1 -> Product/2
  Product/1 -> rw_lat/1, rw_lat x ez/1(a(1) a(2) a(3))
  Selector/1 -> Demux/1

== system mech_motorcycle_stability/Front tire model/Contact/Contact geometry/fw_lat x ez ==
  a(1) a(2) a(3) : Inport  OutDataType=sfix(16)  OutScaling=2^0
  b(1) b(2) b(3) : Inport  Port=2  OutDataType=sfix(16)  OutScaling=2^0
  Product : Product  OutDataType=sfix(16)  OutScaling=2^0  SaturateOnIntegerOverflow=on  RndMeth=Zero  InputSameDT=on  OutDataTypeStr=Inherit: Same as first input
  Product1 : Product  OutDataType=sfix(16)  OutScaling=2^0  SaturateOnIntegerOverflow=on  RndMeth=Zero  InputSameDT=on  OutDataTypeStr=Inherit: Same as first input
  Selector : Selector  InputPortWidth=3  IndexOptions=Index vector (dialog)  Indices=[2 3 1]  OutputSizes=1
  Selector1 : Selector  InputPortWidth=3  IndexOptions=Index vector (dialog)  Indices=[3 1 2]  OutputSizes=1
  Selector2 : Selector  InputPortWidth=3  IndexOptions=Index vector (dialog)  Indices=[2 3 1]  OutputSizes=1
  Selector3 : Selector  InputPortWidth=3  IndexOptions=Index vector (dialog)  Indices=[3 1 2]  OutputSizes=1
  Sum : Sum  Inputs=+|-  OutDataType=sfix(16)  OutScaling=2^0  SaturateOnIntegerOverflow=on  InputSameDT=on  OutDataTypeStr=Inherit: Same as first input
  c(1) c(2) c(3) : Outport  OutDataType=sfix(16)  OutScaling=2^0  InitialOutput=0
  wires:
  Sum/1 -> c(1) c(2) c(3)/1
  b(1) b(2) b(3)/1 -> Selector1/1, Selector2/1
  Selector/1 -> Product/1
  a(1) a(2) a(3)/1 -> Selector/1, Selector3/1
  Product/1 -> Sum/1
  Selector1/1 -> Product/2
  Product1/1 -> Sum/2
  Selector2/1 -> Product1/2
  Selector3/1 -> Product1/1

== system mech_motorcycle_stability/Rear tire model/Contact/Contact geometry/rw_lat x ez ==
  a(1) a(2) a(3) : Inport  OutDataType=sfix(16)  OutScaling=2^0
  b(1) b(2) b(3) : Inport  Port=2  OutDataType=sfix(16)  OutScaling=2^0
  Product : Product  OutDataType=sfix(16)  OutScaling=2^0  SaturateOnIntegerOverflow=on  RndMeth=Zero  InputSameDT=on  OutDataTypeStr=Inherit: Same as first input
  Product1 : Product  OutDataType=sfix(16)  OutScaling=2^0  SaturateOnIntegerOverflow=on  RndMeth=Zero  InputSameDT=on  OutDataTypeStr=Inherit: Same as first input
  Selector : Selector  InputPortWidth=3  IndexOptions=Index vector (dialog)  Indices=[2 3 1]  OutputSizes=1
  Selector1 : Selector  InputPortWidth=3  IndexOptions=Index vector (dialog)  Indices=[3 1 2]  OutputSizes=1
  Selector2 : Selector  InputPortWidth=3  IndexOptions=Index vector (dialog)  Indices=[2 3 1]  OutputSizes=1
  Selector3 : Selector  InputPortWidth=3  IndexOptions=Index vector (dialog)  Indices=[3 1 2]  OutputSizes=1
  Sum : Sum  Inputs=+|-  OutDataType=sfix(16)  OutScaling=2^0  SaturateOnIntegerOverflow=on  InputSameDT=on  OutDataTypeStr=Inherit: Same as first input
  c(1) c(2) c(3) : Outport  OutDataType=sfix(16)  OutScaling=2^0  InitialOutput=0
  wires:
  Sum/1 -> c(1) c(2) c(3)/1
  b(1) b(2) b(3)/1 -> Selector1/1, Selector2/1
  Selector/1 -> Product/1
  a(1) a(2) a(3)/1 -> Selector/1, Selector3/1
  Product/1 -> Sum/1
  Selector1/1 -> Product/2
  Product1/1 -> Sum/2
  Selector2/1 -> Product1/2
  Selector3/1 -> Product1/1
